simulink model "FOC1"  (R2018b)
settings: Solver=VariableStepAuto  StartTime=0.0  StopTime=2  RelTol=1e-3
values from neighbouring files (symbols this model uses):
  B = 0    [FocInit.m]
  Flux = 0.0083333    [FocInit.m]
  J = 2.81e-4    (= 0.000281)    [FocInit.m]
  L = 6e-5    (= 6e-05)    [FocInit.m]
  Pn = 4    [FocInit.m]
  R = 0.003    [FocInit.m]
  Tf = 0    [FocInit.m]
libraries: powerlib x6, simulink x4
settings Model: Creator=ChenZ  LastModifiedBy=ChenZ

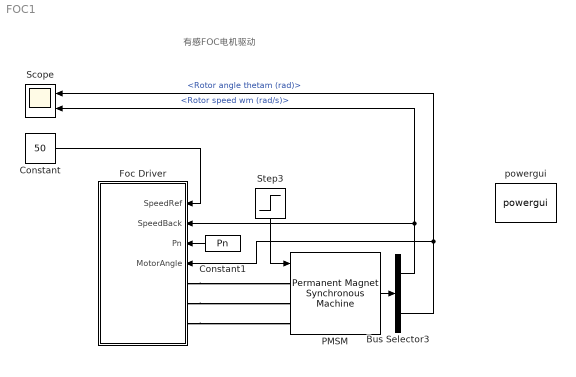
== system FOC1 ==
  note: 有感FOC电机驱动
  Bus Selector3 : BusSelector  OutputSignals=Rotor speed wm (rad/s),Rotor angle thetam (rad)
  Constant : Constant  Value=50
  Constant1 : Constant  Value=Pn
  Foc Driver : Subsystem
  "PMSM " : powerlib/Machines/Permanent Magnet Synchronous Machine  NbPhases=3  FluxDistribution=Sinusoidal  RotorType=Round  MechanicalLoad=Torque Tm  PresetModel=No  ShowDetailedParameters=on  MeasurementBus=off  Resistance=R  Inductance=8.5e-3  dqInductances=[8.5e-3, 8.5e-3]  La=L  MachineConstant=Torque Constant (N.m / A_peak)  Flux=0.0083333  VoltageCst=6.046  TorqueCst=T  Flat=120  Mechanical=[J,B,Pn,Tf]  PolePairs=4  InitialConditions=[0,0, 0,0]  InitialConditions5ph=[0 0 0 0 0 0]  TsPowergui=0  TsBlock=-1  RefAngle=Aligned with phase A axis (original Park)
      settings: SourceProductName=Simscape Power Systems
  Scope : Scope  NumInputPorts=2
  Step3 : Step  Time=0  After=0  SampleTime=0
  powergui : powerlib/powergui  Priority=1  SimulationMode=Discrete  SampleTime=0.000001  frequency=60  Iterations=50  frequencyindice=0  Pbase=100e6  ErrMax=1e-4  UnitsV=kV  UnitsW=MW  buscounter=0  FunctionMessages=off  echomessages=off  EnableUseOfTLC=off  CurrentSourceSwitches=off  DisableSnubberDevices=off  DisableRonSwitches=off  DisableVfSwitches=off  DisplayEquations=off  SolverType=Tustin/Backward Euler (TBE)  Interpol=off  ExternalGateDelay=off  methode=off  Ts=100  x0status=blocks  SPID=off  SwTol=0  HookPort=off  RestoreLinks=warning  ResistiveCurrentMeasurement=off  Frange=[0:2:500]  Ylog=off  Xlog=on  ShowGrid=off  save=off  variable=ZData  structure=0  ZoomFFT=off  StartTime=0.0  cycles=1  DisplayStyle=1  fundamental=60  FreqAxis=off  MaxFrequency=1000  frequencyindicesteady=1  RmsSteady=1  display=off
  wires:
  Bus Selector3/1 -> Scope/2, Foc Driver/2(SpeedBack)  "<Rotor speed wm (rad/s)>"
  Constant/1 -> Foc Driver/1(SpeedRef)
  Bus Selector3/2 -> Scope/1, Foc Driver/4(MotorAngle)  "<Rotor angle thetam (rad)>"
  "PMSM "/1 -> Bus Selector3/1
  Step3/1 -> "PMSM "/1
  Constant1/1 -> Foc Driver/3("Pn ")
  connections:
  Foc Driver/LConn2 -- "PMSM "/LConn2
  Foc Driver/LConn1 -- "PMSM "/LConn1
  Foc Driver/LConn3 -- "PMSM "/LConn3

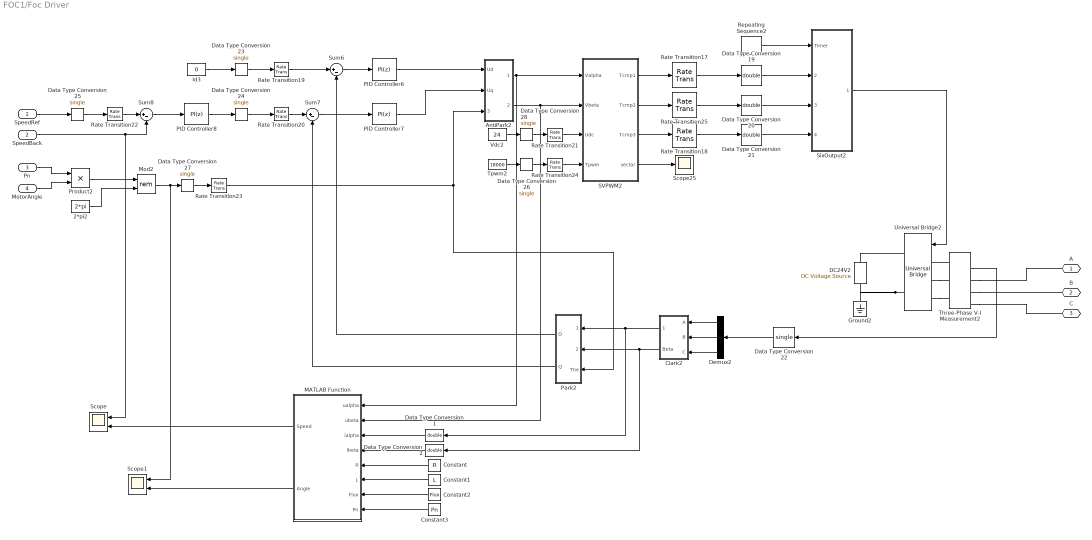
== system FOC1/Foc Driver ==
  SpeedRef : Inport
  SpeedBack : Inport  Port=2
  "Pn " : Inport  Port=3
  MotorAngle : Inport  Port=4
  2*pi2 : Constant  Value=2*pi
  AntiPark2 : Subsystem
  Clark2 : Subsystem
  Constant : Constant  Value=R
  Constant1 : Constant  Value=L
  Constant2 : Constant  Value=Flux
  Constant3 : Constant  Value=Pn
  DC24V2 : powerlib/Electrical Sources/DC Voltage Source  Amplitude=24  Measurements=None
  Data Type Conversion{1..2,19..21} (5 alike) : DataTypeConversion  OutDataTypeStr=double
  Data Type Conversion{22..28} (7 alike) : DataTypeConversion  OutDataTypeStr=single
  Demux2 : Demux  Outputs=3
  Ground2 : powerlib/Elements/Ground  LConnTagsString=a
  Id3 : Constant  Value=0
  MATLAB Function : MATLAB Function  TreatAsAtomicUnit=on
  Mod2 : Math  Operator=rem  SaturateOnIntegerOverflow=on
  PID Controller6 : simulink/Continuous/PID Controller  Controller=PI  Form=Parallel  TimeDomain=Discrete-time  SampleTime=-1  IntegratorMethod=Forward Euler  FilterMethod=Forward Euler  ControllerParametersSource=internal  P=0.2  I=100  D=0  UseFilter=on  N=100  TunerSelectOption=Transfer Function Based (PID Tuner App)  InitialConditionSource=internal  InitialConditionForIntegrator=0  InitialConditionForFilter=0  DifferentiatorICPrevScaledInput=0  ExternalReset=none  TrackingMode=off  Kt=1  LimitOutput=off  UpperSaturationLimit=inf  LowerSaturationLimit=-inf  LinearizeAsGain=on  AntiWindupMode=none  Kb=1  POutMin=[]  POutMax=[]  IOutMin=[]  IOutMax=[]  DOutMin=[]  DOutMax=[]  NOutMin=[]  NOutMax=[]  SumOutMin=[]  SumOutMax=[]  SaturationOutMin=[]  SaturationOutMax=[]  PParamMin=[]  PParamMax=[]  IParamMin=[]  IParamMax=[]  DParamMin=[]  DParamMax=[]  NParamMin=[]  NParamMax=[]  KbParamMin=[]  KbParamMax=[]  KtParamMin=[]  KtParamMax=[]  KbOutMin=[]  KbOutMax=[]  KtOutMin=[]  KtOutMax=[]  IntegratorOutMin=[]  IntegratorOutMax=[]  FilterOutMin=[]  FilterOutMax=[]  SumI1OutMin=[]  SumI1OutMax=[]  SumI2OutMin=[]  SumI2OutMax=[]  SumI3OutMin=[]  SumI3OutMax=[]  SumI4OutMin=[]  SumI4OutMax=[]  SumDOutMin=[]  SumDOutMax=[]  DifferentiatorOutMin=[]  DifferentiatorOutMax=[]  FilterDiffOutCoefMin=[]  FilterDiffOutCoefMax=[]  ReciprocalOutMin=[]  ReciprocalOutMax=[]  SumDenOutMin=[]  SumDenOutMax=[]  SumNumOutMin=[]  SumNumOutMax=[]  DivideOutMin=[]  DivideOutMax=[]  IntegratorContinuousStateAttributes=''  IntegratorStateMustResolveToSignalObject=off  IntegratorRTWStateStorageClass=Auto  FilterContinuousStateAttributes=''  FilterStateMustResolveToSignalObject=off  FilterRTWStateStorageClass=Auto  ParallelPVariant=InternalParameters  IdealPVariant=Disabled  IVariant=InternalParameters  DVariant=Disabled  IntegratorVariant=Discrete  SatVariant=Disabled  AWVariant=Passthrough  PCopyVariant=Disabled  TRVariant=Disabled  FdbkBlocksVariant=Forward  IdealPFdbkVariant=Disabled  SatFdbkVariant=Disabled  DerivativeFilterVariant=Disabled  NVariant=Disabled  NCopyVariant=Disabled_SignalSpec  FilterICVariant=Disabled  IntegratorICVariant=InternalICs  ExternalResetVariant=Disabled  TRSumVariant=Passthrough  SumFdbkVariant=Disabled  SumVariant=Sum_PI
  PID Controller7 : simulink/Continuous/PID Controller  Controller=PI  Form=Parallel  TimeDomain=Discrete-time  SampleTime=-1  IntegratorMethod=Forward Euler  FilterMethod=Forward Euler  ControllerParametersSource=internal  P=0.2  I=100  D=0  UseFilter=on  N=100  TunerSelectOption=Transfer Function Based (PID Tuner App)  InitialConditionSource=internal  InitialConditionForIntegrator=0  InitialConditionForFilter=0  DifferentiatorICPrevScaledInput=0  ExternalReset=none  TrackingMode=off  Kt=1  LimitOutput=off  UpperSaturationLimit=inf  LowerSaturationLimit=-inf  LinearizeAsGain=on  AntiWindupMode=none  Kb=1  POutMin=[]  POutMax=[]  IOutMin=[]  IOutMax=[]  DOutMin=[]  DOutMax=[]  NOutMin=[]  NOutMax=[]  SumOutMin=[]  SumOutMax=[]  SaturationOutMin=[]  SaturationOutMax=[]  PParamMin=[]  PParamMax=[]  IParamMin=[]  IParamMax=[]  DParamMin=[]  DParamMax=[]  NParamMin=[]  NParamMax=[]  KbParamMin=[]  KbParamMax=[]  KtParamMin=[]  KtParamMax=[]  KbOutMin=[]  KbOutMax=[]  KtOutMin=[]  KtOutMax=[]  IntegratorOutMin=[]  IntegratorOutMax=[]  FilterOutMin=[]  FilterOutMax=[]  SumI1OutMin=[]  SumI1OutMax=[]  SumI2OutMin=[]  SumI2OutMax=[]  SumI3OutMin=[]  SumI3OutMax=[]  SumI4OutMin=[]  SumI4OutMax=[]  SumDOutMin=[]  SumDOutMax=[]  DifferentiatorOutMin=[]  DifferentiatorOutMax=[]  FilterDiffOutCoefMin=[]  FilterDiffOutCoefMax=[]  ReciprocalOutMin=[]  ReciprocalOutMax=[]  SumDenOutMin=[]  SumDenOutMax=[]  SumNumOutMin=[]  SumNumOutMax=[]  DivideOutMin=[]  DivideOutMax=[]  IntegratorContinuousStateAttributes=''  IntegratorStateMustResolveToSignalObject=off  IntegratorRTWStateStorageClass=Auto  FilterContinuousStateAttributes=''  FilterStateMustResolveToSignalObject=off  FilterRTWStateStorageClass=Auto  ParallelPVariant=InternalParameters  IdealPVariant=Disabled  IVariant=InternalParameters  DVariant=Disabled  IntegratorVariant=Discrete  SatVariant=Disabled  AWVariant=Passthrough  PCopyVariant=Disabled  TRVariant=Disabled  FdbkBlocksVariant=Forward  IdealPFdbkVariant=Disabled  SatFdbkVariant=Disabled  DerivativeFilterVariant=Disabled  NVariant=Disabled  NCopyVariant=Disabled_SignalSpec  FilterICVariant=Disabled  IntegratorICVariant=InternalICs  ExternalResetVariant=Disabled  TRSumVariant=Passthrough  SumFdbkVariant=Disabled  SumVariant=Sum_PI
  PID Controller8 : simulink/Continuous/PID Controller  Controller=PI  Form=Parallel  TimeDomain=Discrete-time  SampleTime=-1  IntegratorMethod=Forward Euler  FilterMethod=Forward Euler  ControllerParametersSource=internal  P=0.3892  I=3.147  D=0  UseFilter=on  N=100  TunerSelectOption=Transfer Function Based (PID Tuner App)  InitialConditionSource=internal  InitialConditionForIntegrator=0  InitialConditionForFilter=0  DifferentiatorICPrevScaledInput=0  ExternalReset=none  TrackingMode=off  Kt=1  LimitOutput=off  UpperSaturationLimit=inf  LowerSaturationLimit=-inf  LinearizeAsGain=on  AntiWindupMode=none  Kb=1  POutMin=[]  POutMax=[]  IOutMin=[]  IOutMax=[]  DOutMin=[]  DOutMax=[]  NOutMin=[]  NOutMax=[]  SumOutMin=[]  SumOutMax=[]  SaturationOutMin=[]  SaturationOutMax=[]  PParamMin=[]  PParamMax=[]  IParamMin=[]  IParamMax=[]  DParamMin=[]  DParamMax=[]  NParamMin=[]  NParamMax=[]  KbParamMin=[]  KbParamMax=[]  KtParamMin=[]  KtParamMax=[]  KbOutMin=[]  KbOutMax=[]  KtOutMin=[]  KtOutMax=[]  IntegratorOutMin=[]  IntegratorOutMax=[]  FilterOutMin=[]  FilterOutMax=[]  SumI1OutMin=[]  SumI1OutMax=[]  SumI2OutMin=[]  SumI2OutMax=[]  SumI3OutMin=[]  SumI3OutMax=[]  SumI4OutMin=[]  SumI4OutMax=[]  SumDOutMin=[]  SumDOutMax=[]  DifferentiatorOutMin=[]  DifferentiatorOutMax=[]  FilterDiffOutCoefMin=[]  FilterDiffOutCoefMax=[]  ReciprocalOutMin=[]  ReciprocalOutMax=[]  SumDenOutMin=[]  SumDenOutMax=[]  SumNumOutMin=[]  SumNumOutMax=[]  DivideOutMin=[]  DivideOutMax=[]  IntegratorContinuousStateAttributes=''  IntegratorStateMustResolveToSignalObject=off  IntegratorRTWStateStorageClass=Auto  FilterContinuousStateAttributes=''  FilterStateMustResolveToSignalObject=off  FilterRTWStateStorageClass=Auto  ParallelPVariant=InternalParameters  IdealPVariant=Disabled  IVariant=InternalParameters  DVariant=Disabled  IntegratorVariant=Discrete  SatVariant=Disabled  AWVariant=Passthrough  PCopyVariant=Disabled  TRVariant=Disabled  FdbkBlocksVariant=Forward  IdealPFdbkVariant=Disabled  SatFdbkVariant=Disabled  DerivativeFilterVariant=Disabled  NVariant=Disabled  NCopyVariant=Disabled_SignalSpec  FilterICVariant=Disabled  IntegratorICVariant=InternalICs  ExternalResetVariant=Disabled  TRSumVariant=Passthrough  SumFdbkVariant=Disabled  SumVariant=Sum_PI
  Park2 : Subsystem
  Product2 : Product
  Rate Transition{17..25} (9 alike) : RateTransition
  Repeating Sequence2 : simulink/Sources/Repeating Sequence  rep_seq_t=[0 0.00005 0.0001]  rep_seq_y=[0 9000 0]
  SVPWM2 : MATLAB Function  TreatAsAtomicUnit=on
  Scope : Scope  NumInputPorts=2
  Scope1 : Scope  NumInputPorts=2
  Scope25 : Scope
  SixOutput2 : Subsystem
  Sum6 : Sum  Inputs=|+-
  Sum7 : Sum  Inputs=|+-
  Sum8 : Sum  Inputs=|+-
  Three-Phase V-I Measurement2 : powerlib/Measurements/Three-Phase V-I Measurement  VoltageMeasurement=phase-to-ground  SetLabelV=off  LabelV=Vabc  Vpu=off  VpuLL=off  CurrentMeasurement=yes  SetLabelI=off  LabelI=Iabc  Ipu=off  Pbase=100e6  Vbase=500e3  OutputType=Complex  PhasorSimulation=off  PSBequivalent=0
  Tpwm2 : Constant  Value=18000
  Universal Bridge2 : powerlib/Power Electronics/Universal Bridge  Arms=3  SnubberResistance=1e5  SnubberCapacitance=inf  Device=IGBT / Diodes  Ron=1e-3  Lon=0  ForwardVoltages="[  0  0  ]"  ForwardVoltage=0  GTOparameters=[ 10e-6 , 20e-6 ]  IGBTparameters=[ 1e-6 , 2e-6 ]  Measurements=None  Measurements_2=None  converterType=Rectifier
  Vdc2 : Constant  Value=24
  A : PMIOPort  Side=Left
  B : PMIOPort  Port=2  Side=Left
  C : PMIOPort  Port=3  Side=Left
  wires:
  Rate Transition23/1 -> Park2/3(The), AntiPark2/3(theta)
  Sum8/1 -> PID Controller8/1
  SixOutput2/1(drive6) -> Universal Bridge2/1
  Demux2/2 -> Clark2/2(B)
  SVPWM2/3(Tcmp3) -> Rate Transition18/1
  Data Type Conversion28/1 -> Rate Transition21/1
  Rate Transition22/1 -> Sum8/1
  PID Controller8/1 -> Data Type Conversion24/1
  SVPWM2/4(sector) -> Scope25/1
  Data Type Conversion24/1 -> Rate Transition20/1
  SpeedBack/1 -> Scope/1, Sum8/2
  Rate Transition18/1 -> Data Type Conversion21/1
  Data Type Conversion22/1 -> Demux2/1
  Rate Transition19/1 -> Sum6/1
  Sum6/1 -> PID Controller6/1
  Data Type Conversion21/1 -> SixOutput2/4(Tcmp3)
  Data Type Conversion26/1 -> Rate Transition24/1
  Mod2/1 -> Scope1/1, Data Type Conversion27/1
  Sum7/1 -> PID Controller7/1
  MotorAngle/1 -> Product2/2
  PID Controller6/1 -> AntiPark2/1(Ud)
  Demux2/3 -> Clark2/3(C)
  SVPWM2/1(Tcmp1) -> Rate Transition17/1
  Product2/1 -> Mod2/1
  Tpwm2/1 -> Data Type Conversion26/1
  Vdc2/1 -> Data Type Conversion28/1
  Data Type Conversion20/1 -> SixOutput2/3(Tcmp2)
  Demux2/1 -> Clark2/1(A)
  Data Type Conversion25/1 -> Rate Transition22/1
  Data Type Conversion19/1 -> SixOutput2/2(Tcmp1)
  Rate Transition24/1 -> SVPWM2/4(Tpwm)
  Rate Transition17/1 -> Data Type Conversion19/1
  "Pn "/1 -> Product2/1
  SpeedRef/1 -> Data Type Conversion25/1
  Three-Phase V-I Measurement2/2 -> Data Type Conversion22/1
  Park2/2(Q) -> Sum7/2
  Data Type Conversion27/1 -> Rate Transition23/1
  Id3/1 -> Data Type Conversion23/1
  SVPWM2/2(Tcmp2) -> Rate Transition25/1
  Rate Transition25/1 -> Data Type Conversion20/1
  Rate Transition20/1 -> Sum7/1
  2*pi2/1 -> Mod2/2
  Rate Transition21/1 -> SVPWM2/3(Udc)
  PID Controller7/1 -> AntiPark2/2(Uq)
  Repeating Sequence2/1 -> SixOutput2/1(Timer)
  Park2/1(D) -> Sum6/2
  Data Type Conversion23/1 -> Rate Transition19/1
  MATLAB Function/1(Speed) -> Scope/2
  Clark2/1(Alpha) -> Data Type Conversion1/1, Park2/1(Alpha)
  Clark2/2(Beta) -> Data Type Conversion2/1, Park2/2(Beta)
  MATLAB Function/2(Angle) -> Scope1/2
  AntiPark2/1(Ualpha) -> MATLAB Function/1(ualpha), SVPWM2/1(Valpha)
  AntiPark2/2(Ubeta) -> MATLAB Function/2(ubeta), SVPWM2/2(Vbeta)
  Data Type Conversion1/1 -> MATLAB Function/3(ialpha)
  Data Type Conversion2/1 -> MATLAB Function/4(ibeta)
  Constant/1 -> MATLAB Function/5(R)
  Constant1/1 -> MATLAB Function/6(L)
  Constant2/1 -> MATLAB Function/7(Flux)
  Constant3/1 -> MATLAB Function/8(Pn)
  connections:
  Universal Bridge2/RConn2 -- DC24V2/LConn1 -- Ground2/LConn1
  Universal Bridge2/LConn3 -- Three-Phase V-I Measurement2/LConn3
  Universal Bridge2/LConn2 -- Three-Phase V-I Measurement2/LConn2
  Three-Phase V-I Measurement2/RConn1 -- A/RConn1
  DC24V2/RConn1 -- Universal Bridge2/RConn1
  Three-Phase V-I Measurement2/LConn1 -- Universal Bridge2/LConn1
  Three-Phase V-I Measurement2/RConn2 -- B/RConn1
  Three-Phase V-I Measurement2/RConn3 -- C/RConn1

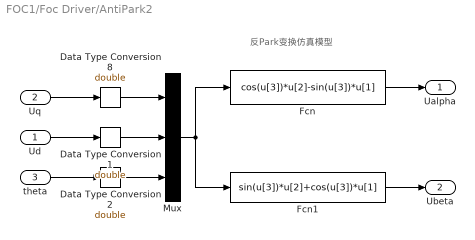
== system FOC1/Foc Driver/AntiPark2 ==
  note: 反Park变换仿真模型
  Ud : Inport
  Uq : Inport  Port=2
  theta : Inport  Port=3
  Data Type Conversion1 : DataTypeConversion  OutDataTypeStr=double
  Data Type Conversion2 : DataTypeConversion  OutDataTypeStr=double
  Data Type Conversion8 : DataTypeConversion  OutDataTypeStr=double
  Fcn : Fcn  Expr=cos(u[3])*u[2]-sin(u[3])*u[1]
  Fcn1 : Fcn  Expr=sin(u[3])*u[2]+cos(u[3])*u[1]
  Mux : Mux  Inputs=3
  Ualpha : Outport
  Ubeta : Outport  Port=2
  wires:
  Mux/1 -> Fcn/1, Fcn1/1
  Fcn/1 -> Ualpha/1
  Fcn1/1 -> Ubeta/1
  theta/1 -> Data Type Conversion2/1
  Data Type Conversion2/1 -> Mux/3
  Data Type Conversion1/1 -> Mux/2
  Ud/1 -> Data Type Conversion1/1
  Uq/1 -> Data Type Conversion8/1
  Data Type Conversion8/1 -> Mux/1

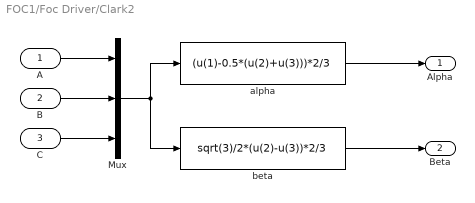
== system FOC1/Foc Driver/Clark2 ==
  A : Inport
  B : Inport  Port=2
  C : Inport  Port=3
  Mux : Mux  Inputs=3
  alpha : Fcn  Expr=(u(1)-0.5*(u(2)+u(3)))*2/3
  beta : Fcn  Expr=sqrt(3)/2*(u(2)-u(3))*2/3
  Alpha : Outport
  Beta : Outport  Port=2
  wires:
  alpha/1 -> Alpha/1
  B/1 -> Mux/2
  C/1 -> Mux/3
  A/1 -> Mux/1
  Mux/1 -> beta/1, alpha/1
  beta/1 -> Beta/1

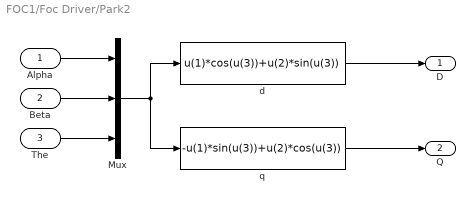
== system FOC1/Foc Driver/Park2 ==
  Alpha : Inport
  Beta : Inport  Port=2
  The : Inport  Port=3
  Mux : Mux  Inputs=3
  d : Fcn  Expr=u(1)*cos(u(3))+u(2)*sin(u(3))
  q : Fcn  Expr=-u(1)*sin(u(3))+u(2)*cos(u(3))
  D : Outport
  Q : Outport  Port=2
  wires:
  d/1 -> D/1
  Beta/1 -> Mux/2
  The/1 -> Mux/3
  Alpha/1 -> Mux/1
  Mux/1 -> q/1, d/1
  q/1 -> Q/1

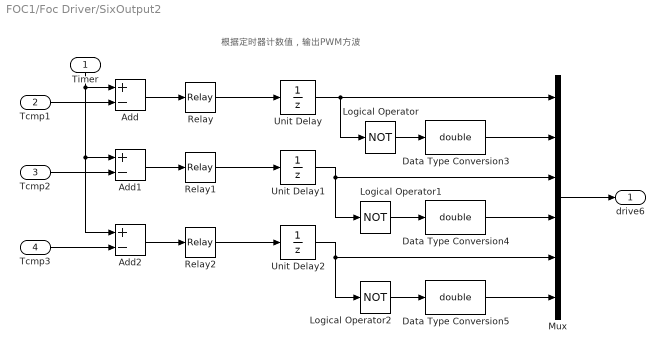
== system FOC1/Foc Driver/SixOutput2 ==
  note: 根据定时器计数值，输出PWM方波
  Timer : Inport
  Tcmp1 : Inport  Port=2
  Tcmp2 : Inport  Port=3
  Tcmp3 : Inport  Port=4
  Add : Sum  Inputs=+-
  Add1 : Sum  Inputs=+-
  Add2 : Sum  Inputs=+-
  Data Type Conversion3 : DataTypeConversion  OutDataTypeStr=double
  Data Type Conversion4 : DataTypeConversion  OutDataTypeStr=double
  Data Type Conversion5 : DataTypeConversion  OutDataTypeStr=double
  Logical Operator : Logic  Operator=NOT  AllPortsSameDT=off  OutDataTypeStr=boolean
  Logical Operator1 : Logic  Operator=NOT  AllPortsSameDT=off  OutDataTypeStr=boolean
  Logical Operator2 : Logic  Operator=NOT  AllPortsSameDT=off  OutDataTypeStr=boolean
  Mux : Mux  Inputs=6
  Relay : Relay  OffSwitchValue=-eps
  Relay1 : Relay  OffSwitchValue=-eps
  Relay2 : Relay  OffSwitchValue=-eps
  Unit Delay : UnitDelay  SampleTime=-1
  Unit Delay1 : UnitDelay  SampleTime=-1
  Unit Delay2 : UnitDelay  SampleTime=-1
  drive6 : Outport
  wires:
  Logical Operator2/1 -> Data Type Conversion5/1
  Unit Delay2/1 -> Mux/5, Logical Operator2/1
  Logical Operator/1 -> Data Type Conversion3/1
  Timer/1 -> Add2/1, Add1/1, Add/1
  Relay2/1 -> Unit Delay2/1
  Add1/1 -> Relay1/1
  Tcmp3/1 -> Add2/2
  Data Type Conversion4/1 -> Mux/4
  Unit Delay1/1 -> Mux/3, Logical Operator1/1
  Relay1/1 -> Unit Delay1/1
  Add/1 -> Relay/1
  Unit Delay/1 -> Logical Operator/1, Mux/1
  Relay/1 -> Unit Delay/1
  Mux/1 -> drive6/1
  Tcmp1/1 -> Add/2
  Data Type Conversion5/1 -> Mux/6
  Add2/1 -> Relay2/1
  Logical Operator1/1 -> Data Type Conversion4/1
  Tcmp2/1 -> Add1/2
  Data Type Conversion3/1 -> Mux/2

== matlab function FOC1/Foc Driver/MATLAB Function ==
  data: ualpha input; Speed output; ubeta input; ialpha input; ibeta input; R input; L input; Flux input; Angle output; Pn input
function [Speed,Angle] = EKF(ualpha,ubeta,ialpha,ibeta,R,L,Flux,Pn)
persistent Flag x Pm;
%1、进行数据初始化
if isempty(Flag)
    Flag = 1;
    %初始化状态向量
    x=zeros(4,1);
    %定义协方差矩阵
    Pm=diag([0 0 0 0]);
end
%2、定义过程噪声协方差矩阵
Qm=[0.001,0,0,0; 0,0.001,0,0; 0,0,0.001,0; 0,0,0,0.001];
%3、定义观测噪声协方差矩阵
Rm=[0.001,0; 0,0.001];
%4、定义相邻两次卡尔曼滤波运行间隔时间
Ts=1e-6;
%5、定义系统矩阵
Am=[-R/L,0,Flux/L*sin(x(4)),Flux/L*x(3)*cos(x(4));
           0,-R/L,-Flux/L*cos(x(4)),Flux/L*x(3)*sin(x(4));
           0,0,1,0;
           0,0,1,1];
%2、定义输入矩阵
Bm=[1.0/L,0; 0,1.0/L; 0,0; 0,0];
%3、定义观测矩阵
Hm=eye(2,4);
%4、定义非线性矩阵
Fm=[-R/L*x(1)+Flux/L*x(3)*sin(x(4));
         -R/L*x(2)-Flux/L*x(3)*cos(x(4));
         0
         x(3)];
%5、离散化模型
AmHat=eye(4)+Ts*Am;
BmHat=Ts*Bm;
FmHat=Ts*Fm;
%6、读取输入变量
u=[ualpha;ubeta];
%7、读取测量变量
z=[ialpha;ibeta];
% ------------ 预测步骤 ------------
%8、状态预测
xHat=x+FmHat+BmHat*u;
%9、测量变量的预测
zHat=Hm*xHat;
%10、协方差预测
PmHat=AmHat*Pm*AmHat'+Qm;
% ------------ 更新步骤 ------------
%11、计算卡尔曼增益
Km=PmHat*Hm'/(Hm*PmHat*Hm'+Rm);
%12、更新状态变量       
x=xHat+Km*(z-zHat);
%13、协方差更新
Pm=(eye(4)-Km*Hm)*PmHat;
%14、电机转速和电转角的输出
Speed=x(3)/Pn;
Angle=rem(x(4),2*pi);
end

== matlab function FOC1/Foc Driver/SVPWM2 ==
  data: Valpha input; Tcmp1 output; Vbeta input; Udc input; Tpwm input; Tcmp2 output; Tcmp3 output; sector output
%输入变量：电压Ualpha、电压Ubeta、驱动器直流供电电压Udc、输出PWM波形的周期计数值
%输出变量：扇区、输出波形1、输出波形2、输出波形3
function [Tcmp1,Tcmp2,Tcmp3,sector] = fcn(Valpha,Vbeta,Udc,Tpwm)

%初始化输出变量：扇区、输出波形1、输出波形2、输出波形3
sector = single(0);
sectorTemp = single(0);
Tcmp1 = single(0);
Tcmp2 = single(0);
Tcmp3 = single(0);

%定义扇区三个判据表达式
Vref1 = Vbeta;							                   
Vref2 = (sqrt(3)*Valpha - Vbeta)/2; 				    
Vref3 = (-sqrt(3)*Valpha - Vbeta)/2;					
%计算扇区判据
%sector：1   2   3   4   5   6
%判据：    3   1   5   4   6   2
if (Vref1>0)
    sectorTemp = single(1);
end
if (Vref2>0)
    sectorTemp = sectorTemp+single(2);
end
if (Vref3>0)
	sectorTemp = sectorTemp+single(4);
end

%定义矢量合成作用时间的三个表达式判据
X = sqrt(3)*Vbeta*Tpwm/Udc;
Y = Tpwm/Udc*(3/2*Valpha+sqrt(3)/2*Vbeta);
Z = Tpwm/Udc*(-3/2*Valpha+sqrt(3)/2*Vbeta);	         
%计算占空比
switch (sectorTemp)   
    case 1
        T1 = Z; T2 = Y; 
	case 2
        T1 = Y; T2 = -X; 
	case 3
        T1 = -Z; T2 = X; 
	case 4
        T1 = -X; T2 = Z;
	case 5
        T1 = X; T2 = -Y;
    otherwise
        T1 = -Y; T2 = -Z;
end

if T1+T2 > Tpwm
    T1 = T1/(T1+T2);
    T2 = T2/(T1+T2);
else
    T1 = T1;
    T2 = T2;
end

%计算输出定时器计数值
ta = (Tpwm-(T1+T2))/4.0;
tb = ta+T1/2;
tc = tb+T2/2;
switch (sectorTemp)
    case 1 
        Tcmp1=tb;
        Tcmp2=ta;
        Tcmp3=tc; 
        sector = single(2);
    case 2 
        Tcmp1=ta;
        Tcmp2=tc;
        Tcmp3=tb;   
        sector = single(6);
    case 3 
        Tcmp1=ta;
        Tcmp2=tb;
        Tcmp3=tc;
        sector = single(1);
    case 4 
        Tcmp1=tc;
        Tcmp2=tb;
        Tcmp3=ta;   
        sector = single(4);
    case 5 
        Tcmp1=tc;
        Tcmp2=ta;
        Tcmp3=tb;
        sector = single(3);
   case 6
       Tcmp1=tb;
       Tcmp2=tc;
       Tcmp3=ta;
       sector = single(5);
end
end
